simulink library "cctc"  (Simulink 8.1)
settings: Solver=ode1  StartTime=0.0  StopTime=Inf  FixedStep=0.001  RelTol=1e-3
PostLoadFcn:
  | , if any(exist('dsrtsu_mdlpostloadfcn', 'file') == [2, 3, 6]), try dsrtsu_mdlpostloadfcn('Execute', bdroot); catch fprintf('Error in PostLoadFcn (dsrtsu_mdlpostloadfcn) for model "%s":\n %s\n', bdroot, lasterr); end, end,
undefined symbols (not defined in the file or in its folder): ENUM_ACCSTATE_DISABLED, FALSE, KJUD_ACCMaxTimeGap_s, KJUD_ACCMediumTimeGap_s, KJUD_ACCMinTimeGap_s, KJUD_ACCNumOfTimeGaps_pos, KJUD_ACCShortTimeGap_s, TRUE
libraries: hcu_lib x1
settings Model: DSRTSU_INTERNAL_RTI_VER=450  DSRTSU_INTERNAL_RTI_TYPE=rti1401  RTICANMMDATA=struct('GeneralSetupData',struct('modelroot','D:\ELN150201_TAIWAN\trunk\AdasDragon\software\sw_development\arch\app\jud','generalsettings',struct('filesettings',struct('destfolder',struct('Name','RTICANMM_FILES','Check',1),'buildfolder',struct('Name','.','Check',1),'AbsDestfolder',struct('Name','D:\ELN150201_TAIWAN\trunk\AdasDragon\software\sw_development\arch\app\jud\RTICANMM_FILES'),'AbsBuildfolder',struct('Name','D:\ELN150201_TAIWAN\trunk\AdasDragon\software\sw_development\arch\app\jud'))),'options',struct('addpaths',1,'rmpaths',1,'addtrcexclusion',logical(1),'cannavigator',struct('checkmonitoring',0),'show_usrtrc',0,'use_usrtrc',0),'advanced',struct('options',[1 1 1 1 1 1 1 1 1 1 1 1 1 1 1 1 1 1 1 1 1 1 1 1 1 1 1 1 1 1 1 1 1 1 1 1 1 1 1 1 1 1 1 1 1 1 1 1 1 1 1 1 1 1 1 1 1 1 1 1 1 1 1 1 1 1 1 1 1 1 1 1 1 1 1 1 1 1 1 1 1 1 1 1 1 1 1 1 1 1 1 1 1 1 1 1 1 1 1 1]),'MPSetup',{{}},'modelname','cctc','block','cctc'))  DSRTSU_INTERNAL_RTIFPGA=40  Creator=AT015411  LastModifiedBy=AT015555

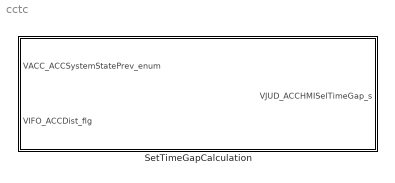
== system cctc ==
  SetTimeGapCalculation : Subsystem

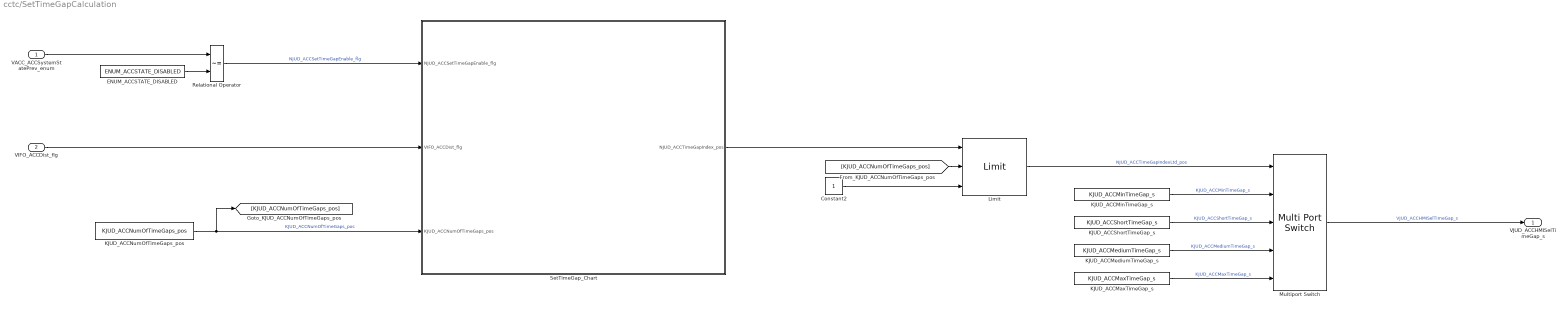
== system cctc/SetTimeGapCalculation ==
  VACC_ACCSystemStatePrev_enum : Inport
  VIFO_ACCDist_flg : Inport  Port=2
  Constant2 : Constant
  ENUM_ACCSTATE_DISABLED : Constant  Value=ENUM_ACCSTATE_DISABLED
  KJUD_ACCMaxTimeGap_s : Constant  Value=KJUD_ACCMaxTimeGap_s
  KJUD_ACCMediumTimeGap_s : Constant  Value=KJUD_ACCMediumTimeGap_s
  KJUD_ACCMinTimeGap_s : Constant  Value=KJUD_ACCMinTimeGap_s
  KJUD_ACCNumOfTimeGaps_pos : Constant  Value=KJUD_ACCNumOfTimeGaps_pos
  KJUD_ACCShortTimeGap_s : Constant  Value=KJUD_ACCShortTimeGap_s
  Limit : hcu_lib/Limit  SystemSampleTime=-1
  Multiport Switch : MultiPortSwitch  Inputs=4  DiagnosticForDefault=None
  Relational Operator : RelationalOperator  Operator=~=  OutDataTypeStr=boolean
  SetTimeGap_Chart : Stateflow chart  TreatAsAtomicUnit=on
  VJUD_ACCHMISelTimeGap_s : Outport
  wires:
  Limit/1 -> Multiport Switch/1  "NJUD_ACCTimeGapIndexLtd_pos"
  Constant2/1 -> Limit/3
  KJUD_ACCMaxTimeGap_s/1 -> Multiport Switch/5  "KJUD_ACCMaxTimeGap_s"
  KJUD_ACCNumOfTimeGaps_pos/1 -> [KJUD_ACCNumOfTimeGaps_pos], SetTimeGap_Chart/3(KJUD_ACCNumOfTimeGaps_pos)  "KJUD_ACCNumOfTimeGaps_pos"
  Multiport Switch/1 -> VJUD_ACCHMISelTimeGap_s/1  "VJUD_ACCHMISelTimeGap_s"
  VIFO_ACCDist_flg/1 -> SetTimeGap_Chart/2(VIFO_ACCDist_flg)
  SetTimeGap_Chart/1(NJUD_ACCTimeGapIndex_pos) -> Limit/1
  KJUD_ACCShortTimeGap_s/1 -> Multiport Switch/3  "KJUD_ACCShortTimeGap_s"
  [KJUD_ACCNumOfTimeGaps_pos] -> Limit/2
  KJUD_ACCMediumTimeGap_s/1 -> Multiport Switch/4  "KJUD_ACCMediumTimeGap_s"
  VACC_ACCSystemStatePrev_enum/1 -> Relational Operator/1
  Relational Operator/1 -> SetTimeGap_Chart/1(NJUD_ACCSetTimeGapEnable_flg)  "NJUD_ACCSetTimeGapEnable_flg"
  KJUD_ACCMinTimeGap_s/1 -> Multiport Switch/2  "KJUD_ACCMinTimeGap_s"
  ENUM_ACCSTATE_DISABLED/1 -> Relational Operator/2

== stateflow chart Untitled ==
  state INITIALIZATION
    en:
    NJUD_ACCTimeGapIndex_pos = KJUD_ACCNumOfTimeGaps_pos;
  state HMI_TGAP
    state HOLD
    state SET_MAX_TGAP
      en:
      NJUD_ACCTimeGapIndex_pos = KJUD_ACCNumOfTimeGaps_pos;
    state DECREASE_GAP
      en:
      NJUD_ACCTimeGapIndex_pos = NJUD_ACCTimeGapIndex_pos-1;
    (default) -> HOLD
    HOLD -> DECREASE_GAP [order 2] : [VIFO_ACCDist_flg == TRUE...
        | && NJUD_ACCTimeGapIndex_pos != 1]
    DECREASE_GAP -> HOLD : [VIFO_ACCDist_flg == FALSE]
    HOLD -> SET_MAX_TGAP [order 1] : [VIFO_ACCDist_flg == TRUE...
        | && NJUD_ACCTimeGapIndex_pos == 1]
    SET_MAX_TGAP -> HOLD : [VIFO_ACCDist_flg == FALSE]
  (default) -> INITIALIZATION
  INITIALIZATION -> HMI_TGAP : [NJUD_ACCSetTimeGapEnable_flg == TRUE]
  HMI_TGAP -> INITIALIZATION : [NJUD_ACCSetTimeGapEnable_flg == FALSE]
  data: NJUD_ACCSetTimeGapEnable_flg input double; VIFO_ACCDist_flg input double; NJUD_ACCTimeGapIndex_pos output single =KJUD_ACCNumOfTimeGaps_pos; TRUE parameter boolean; KJUD_ACCNumOfTimeGaps_pos input double; FALSE parameter boolean
